simulink model "controle_deslizante_full"  (R2018a)
settings: Solver=VariableStepAuto  StartTime=0.0  StopTime=8  MaxStep=0.01  RelTol=1e-3
undefined symbols (not defined in the file): sigbuilder_block
libraries: simulink x1
settings Model: Creator=Mateus Gilbert  LastModifiedBy=renan
settings DataIOCC: ReturnWorkspaceOutputs=on
settings SFSimCC: SimUseLocalCustomCode=on
settings RTWCC: RTWUseLocalCustomCode=on
settings CodeAppCC: StateflowObjectComments=on

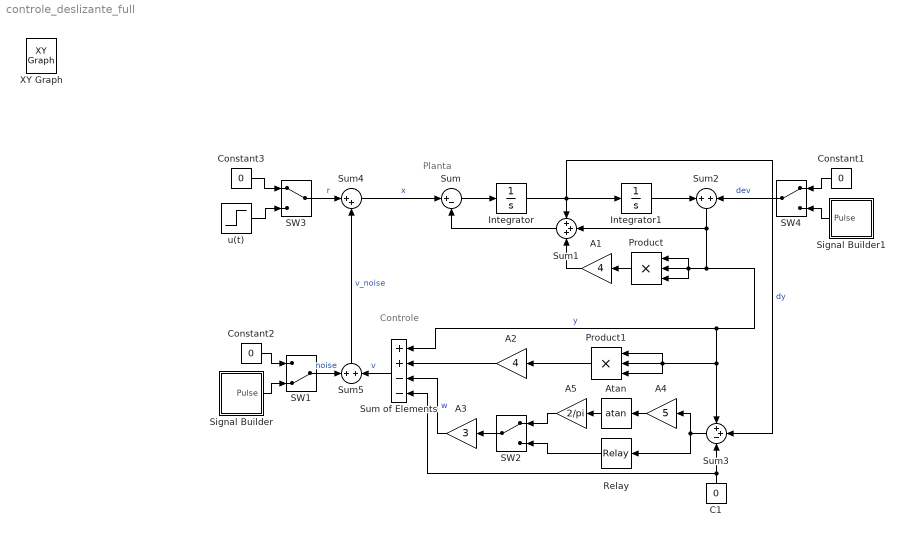
== system controle_deslizante_full ==
  note: Planta
  note: Controle
  A1 : Gain  Gain=4
  A2 : Gain  Gain=4
  A3 : Gain  Gain=3
  A4 : Gain  Gain=5
  A5 : Gain  Gain=2/pi
  Atan : Trigonometry  Operator=atan
  C1 : Constant  Value=0
  Constant1 : Constant  Value=0
  Constant2 : Constant  Value=0
  Constant3 : Constant  Value=0
  Integrator : Integrator  InitialCondition=0.5
  Integrator1 : Integrator  InitialCondition=0.5
  Product : Product  Inputs=3
  Product1 : Product  Inputs=3
  Relay : Relay  OnSwitchValue=1e-5  OffSwitchValue=-1e-5  OffOutputValue=-1
  SW1 : ManualSwitch  CurrentSetting=0
  SW2 : ManualSwitch
  SW3 : ManualSwitch
  SW4 : ManualSwitch
  Signal Builder : Subsystem  Tag=STV Subsys  LoadFcn=sigbuilder_block('load');  StartFcn=sigbuilder_block('start');  StopFcn=sigbuilder_block('stop');  ClipboardFcn=sigbuilder_block('clipboard');  mask(Sigbuilder block){tuvar=[0:10]}
      mask help: Simulink:masks:SigbuilderBlock_MD
      mask init:
      | if ~strcmp(get_param(bdroot(gcbh),'SimulationStatus'),'stopped') tuvar = sigbuilder_block('maskInit'); end
      settings: CopyFcn=sigbuilder_block('copy');  DeleteFcn=sigbuilder_block('delete');  ModelCloseFcn=sigbuilder_block('modelClose');  PreSaveFcn=sigbuilder_block('preSave');  PauseFcn=sigbuilder_block('pause');  ContinueFcn=sigbuilder_block('continue');  NameChangeFcn=sigbuilder_block('namechange');  OpenFcn=sigbuilder_block('open',[280.8 52.2 718.2 400.2 ]);  CloseFcn=sigbuilder_block('close');
      mask Display: plot(0, 0, 100, 100,[2, 2, 32, 32, 2], [68, 8, 8, 68, 68],[32, 2], [38, 38], [32, 19, 2],[53, 60, 44], [32, 17, 17, 2],[16, 16, 31, 31]);txt = getActiveGroup(gcbh);text(2, 100, txt,'verticalAlignment', 'top');
  Signal Builder1 : Subsystem  Tag=STV Subsys  LoadFcn=sigbuilder_block('load');  StartFcn=sigbuilder_block('start');  StopFcn=sigbuilder_block('stop');  ClipboardFcn=sigbuilder_block('clipboard');  mask(Sigbuilder block){tuvar=[0:10]}
      mask help: Simulink:masks:SigbuilderBlock_MD
      mask init:
      | if ~strcmp(get_param(bdroot(gcbh),'SimulationStatus'),'stopped') tuvar = sigbuilder_block('maskInit'); end
      settings: CopyFcn=sigbuilder_block('copy');  DeleteFcn=sigbuilder_block('delete');  ModelCloseFcn=sigbuilder_block('modelClose');  PreSaveFcn=sigbuilder_block('preSave');  PauseFcn=sigbuilder_block('pause');  ContinueFcn=sigbuilder_block('continue');  NameChangeFcn=sigbuilder_block('namechange');  OpenFcn=sigbuilder_block('open',[280.8 52.2 718.2 400.2 ]);  CloseFcn=sigbuilder_block('close');
      mask Display: plot(0, 0, 100, 100,[2, 2, 32, 32, 2], [68, 8, 8, 68, 68],[32, 2], [38, 38], [32, 19, 2],[53, 60, 44], [32, 17, 17, 2],[16, 16, 31, 31]);txt = getActiveGroup(gcbh);text(2, 100, txt,'verticalAlignment', 'top');
  Sum : Sum  Inputs=|+-
  Sum of Elements : Sum  Inputs=++--
  Sum1 : Sum  Inputs=+++
  Sum2 : Sum  Inputs=+|+
  Sum3 : Sum  Inputs=++-
  Sum4 : Sum  Inputs=|++
  Sum5 : Sum  Inputs=+|+
  u(t) : Step  Time=5  SampleTime=0
  XY Graph : simulink/Sinks/XY Graph  IOType=viewer  xmin=-1  xmax=1  ymin=-1  ymax=1  st=-1
  wires:
  Sum/1 -> Integrator/1
  Sum1/1 -> Sum/2
  Product1/1 -> A2/1
  Sum3/1 -> A4/1, Relay/1
  Integrator/1 -> Integrator1/1, Sum3/2, Sum1/1  "dy"
  Sum2/1 -> Sum of Elements/1, Sum3/1, Product1/3, Product1/1, Product1/2, Product/3, Product/1, Product/2, Sum1/2  "y"
  Product/1 -> A1/1
  A1/1 -> Sum1/3
  A2/1 -> Sum of Elements/2
  A3/1 -> Sum of Elements/3  "w"
  Relay/1 -> SW2/2
  SW2/1 -> A3/1
  A4/1 -> Atan/1
  Constant2/1 -> SW1/1
  Signal Builder/1(Pulse) -> SW1/2
  Sum4/1 -> Sum/1  "x"
  SW1/1 -> Sum5/1  "noise"
  Atan/1 -> A5/1
  A5/1 -> SW2/1
  Sum of Elements/1 -> Sum5/2  "v"
  C1/1 -> Sum3/3, Sum of Elements/4
  Integrator1/1 -> Sum2/1
  Constant1/1 -> SW4/1
  SW4/1 -> Sum2/2  "dev"
  Signal Builder1/1(Pulse) -> SW4/2
  SW3/1 -> Sum4/1  "r"
  u(t)/1 -> SW3/2
  Constant3/1 -> SW3/1
  Sum5/1 -> Sum4/2  "v_noise"

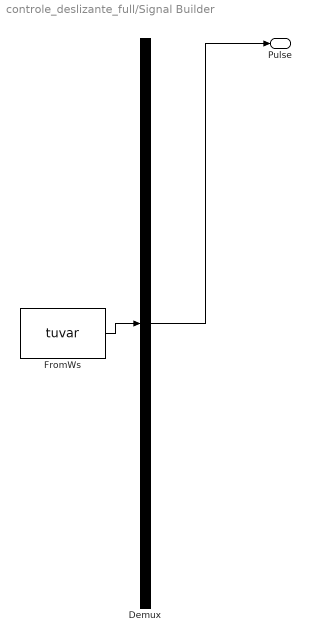
== system controle_deslizante_full/Signal Builder ==
  Demux : Demux  Tag=STV Demux  Outputs=1
  FromWs : FromWorkspace  Tag=STV FromWs  VariableName=tuvar  SampleTime=0
      SigBuilderData=|
      | common.afterFinalStr = 'Extrapolate'
      | common.sampleTime = 0
      | dataSet.timeRange = [0 15]
      | dataSet.name = 'G1'
      | sbobj.Groups.Name = 'G1'
      | sbobj.Groups.Signals.Name = 'Pulse'
      | sbobj.Groups.Signals.XData = [0 4 4 5 5 15]
      | sbobj.Groups.Signals.YData = [0 0 0.4 0.4 0 0]
      | sbobj.Groups.TimeRange = [0 15]
  Pulse : Outport  Tag=STV Outport
  wires:
  Demux/1 -> Pulse/1
  FromWs/1 -> Demux/1

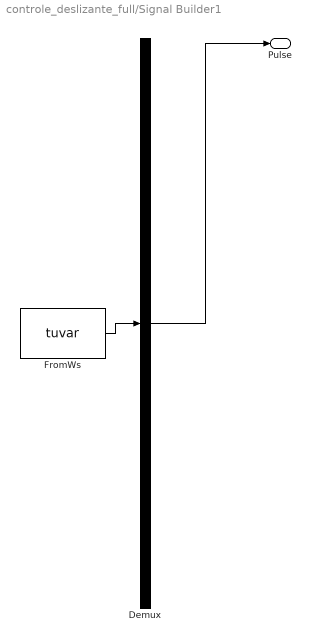
== system controle_deslizante_full/Signal Builder1 ==
  Demux : Demux  Tag=STV Demux  Outputs=1
  FromWs : FromWorkspace  Tag=STV FromWs  VariableName=tuvar  SampleTime=0
      SigBuilderData=|
      | common.afterFinalStr = 'Extrapolate'
      | common.sampleTime = 0
      | dataSet.timeRange = [0 15]
      | dataSet.name = 'G2'
      | sbobj.Groups.Name = 'G2'
      | sbobj.Groups.Signals.Name = 'Pulse'
      | sbobj.Groups.Signals.XData = [0 10 10 12 12 15]
      | sbobj.Groups.Signals.YData = [0 0 2 2 0 0]
      | sbobj.Groups.TimeRange = [0 15]
  Pulse : Outport  Tag=STV Outport
  wires:
  Demux/1 -> Pulse/1
  FromWs/1 -> Demux/1
